simulink model "paper1_inner_loop"  (Simulink 6.0)
settings: Solver=ode45  StartTime=0.0  StopTime=10.0  RelTol=1e-3
values from neighbouring files (symbols this model uses):
  bp = 0.0    (= 0)    [paper1_data.m]
  bt = 0.8    [paper1_data.m]
  Td = 3.36    [paper1_data.m]
  Ti = 0.05    [paper1_data.m]
settings Model: LastModifiedBy=Administrator

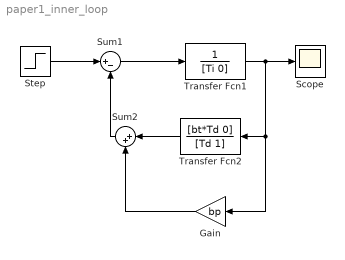
== system paper1_inner_loop ==
  Gain : Gain  Orientation=left  Gain=bp
  Scope : Scope
  Step : Step  SampleTime=0
  Sum1 : Sum  Inputs=|+-
  Sum2 : Sum  Orientation=left  Inputs=|++
  Transfer Fcn1 : TransferFcn  Denominator=[Ti 0]
  Transfer Fcn2 : TransferFcn  Orientation=left  Numerator=[bt*Td 0]  Denominator=[Td 1]
  wires:
  Transfer Fcn1/1 -> Transfer Fcn2/1, Gain/1, Scope/1
  Sum1/1 -> Transfer Fcn1/1
  Gain/1 -> Sum2/2
  Transfer Fcn2/1 -> Sum2/1
  Sum2/1 -> Sum1/2
  Step/1 -> Sum1/1
